simulink model "Project_SADC"  (R2021b)
settings: Solver=ode45  StartTime=0.0  StopTime=T  FixedStep=1e-6  RelTol=1e-12
values from neighbouring files (symbols this model uses):
  A = [A_sc,A_sp]    [Main_SADC_10572571.m]
  Abn0 = Anb0'    [Main_SADC_10572571.m]
  epsilon = deg2rad(23.45)    [Main_SADC_10572571.m]
  m = [0.01 0.05 0.01]'    [Main_SADC_10572571.m]
  N = [n1 n2 n3 n4 n5 n6 n7 n8 n9 n10]    [Main_SADC_10572571.m]
  n_sun = 2*pi / T_sun    (= 1.99238499086e-07)    [Main_SADC_10572571.m]
  P_srp = Fe_tot/c    [Main_SADC_10572571.m]
  R3H0 = data.Re^3*H0    [Main_SADC_10572571.m]
  R_sun = astroConstants(2)    [Main_SADC_10572571.m]
  rho_d = cat(2,ones(1,6)*rho_d_sc,ones(1,4)*rho_d_sp)    [Main_SADC_10572571.m]
  rho_s = cat(2,ones(1,6)*rho_s_sc,ones(1,4)*rho_s_sp)    [Main_SADC_10572571.m]
  ri = [ri_sc,r_sp1,r_sp1,r_sp2,r_sp2]    [Main_SADC_10572571.m]
  w0 = [wx0 wy0 wz0]'    [Main_SADC_10572571.m]
  weights = [0.15;0.5;0.35]    [Main_SADC_10572571.m]
undefined symbols (not defined in the file or in its folder): data, gyro, horizonsensor, magnetometer, rr0, sc, sunsensor, vv0, wheel
libraries: simulink_extras x10
(part 3 of 3)

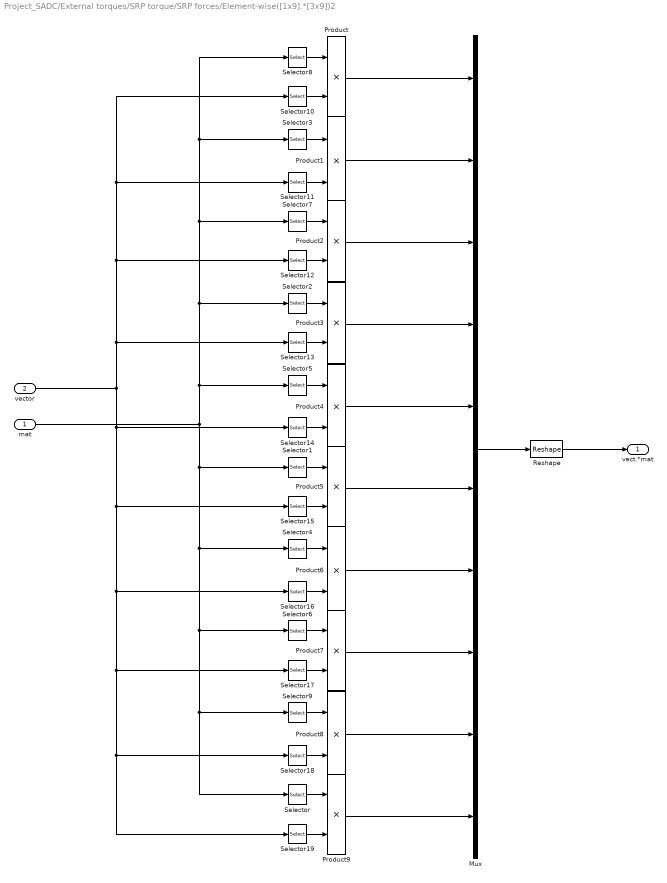
== system Project_SADC/External torques/SRP torque/SRP forces/Element-wise([1x9].*[3x9])2 ==
  mat : Inport
  vector : Inport  Port=2
  Mux : Mux  Inputs=10
  Product{,1..9} (10 alike) : Product
  Reshape : Reshape  OutputDimensionality=Customize  OutputDimensions=[3,10]
  Selector : Selector  NumberOfDimensions=2  InputPortWidth=3  IndexOptions=Index vector (dialog),Index vector (dialog)  Indices=[1 2 3],10  OutputSizes=1,1
  Selector1 : Selector  NumberOfDimensions=2  InputPortWidth=3  IndexOptions=Index vector (dialog),Index vector (dialog)  Indices=[1 2 3],6  OutputSizes=1,1
  Selector10 : Selector  InputPortWidth=10  IndexOptions=Index vector (dialog)  Indices=1  OutputSizes=1
  Selector11 : Selector  InputPortWidth=10  IndexOptions=Index vector (dialog)  Indices=2  OutputSizes=1
  Selector12 : Selector  InputPortWidth=10  IndexOptions=Index vector (dialog)  Indices=3  OutputSizes=1
  Selector13 : Selector  InputPortWidth=10  IndexOptions=Index vector (dialog)  Indices=4  OutputSizes=1
  Selector14 : Selector  InputPortWidth=10  IndexOptions=Index vector (dialog)  Indices=5  OutputSizes=1
  Selector15 : Selector  InputPortWidth=10  IndexOptions=Index vector (dialog)  Indices=6  OutputSizes=1
  Selector16 : Selector  InputPortWidth=10  IndexOptions=Index vector (dialog)  Indices=7  OutputSizes=1
  Selector17 : Selector  InputPortWidth=10  IndexOptions=Index vector (dialog)  Indices=8  OutputSizes=1
  Selector18 : Selector  InputPortWidth=10  IndexOptions=Index vector (dialog)  Indices=9  OutputSizes=1
  Selector19 : Selector  InputPortWidth=10  IndexOptions=Index vector (dialog)  Indices=10  OutputSizes=1
  Selector2 : Selector  NumberOfDimensions=2  InputPortWidth=3  IndexOptions=Index vector (dialog),Index vector (dialog)  Indices=[1 2 3],4  OutputSizes=1,1
  Selector3 : Selector  NumberOfDimensions=2  InputPortWidth=3  IndexOptions=Index vector (dialog),Index vector (dialog)  Indices=[1 2 3],2  OutputSizes=1,1
  Selector4 : Selector  NumberOfDimensions=2  InputPortWidth=3  IndexOptions=Index vector (dialog),Index vector (dialog)  Indices=[1 2 3],7  OutputSizes=1,1
  Selector5 : Selector  NumberOfDimensions=2  InputPortWidth=3  IndexOptions=Index vector (dialog),Index vector (dialog)  Indices=[1 2 3],5  OutputSizes=1,1
  Selector6 : Selector  NumberOfDimensions=2  InputPortWidth=3  IndexOptions=Index vector (dialog),Index vector (dialog)  Indices=[1 2 3],8  OutputSizes=1,1
  Selector7 : Selector  NumberOfDimensions=2  InputPortWidth=3  IndexOptions=Index vector (dialog),Index vector (dialog)  Indices=[1 2 3],3  OutputSizes=1,1
  Selector8 : Selector  NumberOfDimensions=2  InputPortWidth=3  IndexOptions=Index vector (dialog),Index vector (dialog)  Indices=[1 2 3],1  OutputSizes=1,1
  Selector9 : Selector  NumberOfDimensions=2  InputPortWidth=3  IndexOptions=Index vector (dialog),Index vector (dialog)  Indices=[1 2 3],9  OutputSizes=1,1
  vect.*mat : Outport
  wires:
  Product/1 -> Mux/1
  Product1/1 -> Mux/2
  Product2/1 -> Mux/3
  Product3/1 -> Mux/4
  Product4/1 -> Mux/5
  Product6/1 -> Mux/7
  Product5/1 -> Mux/6
  Product7/1 -> Mux/8
  Product8/1 -> Mux/9
  Product9/1 -> Mux/10
  Selector3/1 -> Product1/1
  Selector11/1 -> Product1/2
  Selector7/1 -> Product2/1
  Selector12/1 -> Product2/2
  Selector2/1 -> Product3/1
  Selector13/1 -> Product3/2
  Selector5/1 -> Product4/1
  Selector14/1 -> Product4/2
  Selector1/1 -> Product5/1
  Selector15/1 -> Product5/2
  Selector4/1 -> Product6/1
  Selector16/1 -> Product6/2
  Selector6/1 -> Product7/1
  Selector17/1 -> Product7/2
  Selector18/1 -> Product8/2
  Selector9/1 -> Product8/1
  Selector19/1 -> Product9/2
  Selector/1 -> Product9/1
  Selector10/1 -> Product/2
  Selector8/1 -> Product/1
  vector/1 -> Selector10/1, Selector11/1, Selector12/1, Selector13/1, Selector14/1, Selector15/1, Selector16/1, Selector17/1, Selector18/1, Selector19/1
  mat/1 -> Selector9/1, Selector/1, Selector6/1, Selector4/1, Selector1/1, Selector8/1, Selector3/1, Selector7/1, Selector2/1, Selector5/1
  Reshape/1 -> vect.*mat/1
  Mux/1 -> Reshape/1

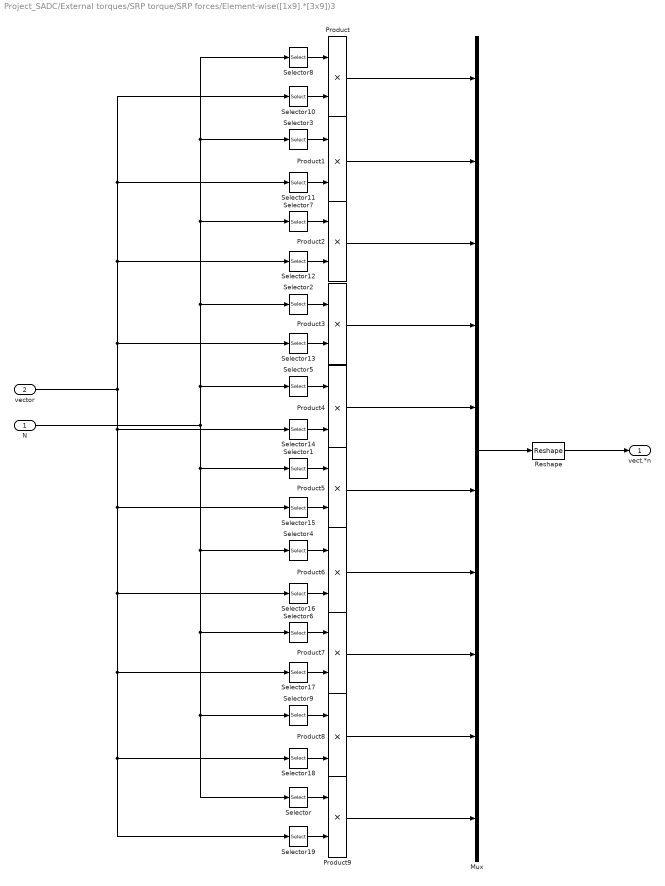
== system Project_SADC/External torques/SRP torque/SRP forces/Element-wise([1x9].*[3x9])3 ==
  N : Inport
  vector : Inport  Port=2
  Mux : Mux  Inputs=10
  Product{,1..9} (10 alike) : Product
  Reshape : Reshape  OutputDimensionality=Customize  OutputDimensions=[3,10]
  Selector : Selector  NumberOfDimensions=2  InputPortWidth=3  IndexOptions=Index vector (dialog),Index vector (dialog)  Indices=[1 2 3],10  OutputSizes=1,1
  Selector1 : Selector  NumberOfDimensions=2  InputPortWidth=3  IndexOptions=Index vector (dialog),Index vector (dialog)  Indices=[1 2 3],6  OutputSizes=1,1
  Selector10 : Selector  InputPortWidth=10  IndexOptions=Index vector (dialog)  Indices=1  OutputSizes=1
  Selector11 : Selector  InputPortWidth=10  IndexOptions=Index vector (dialog)  Indices=2  OutputSizes=1
  Selector12 : Selector  InputPortWidth=10  IndexOptions=Index vector (dialog)  Indices=3  OutputSizes=1
  Selector13 : Selector  InputPortWidth=10  IndexOptions=Index vector (dialog)  Indices=4  OutputSizes=1
  Selector14 : Selector  InputPortWidth=10  IndexOptions=Index vector (dialog)  Indices=5  OutputSizes=1
  Selector15 : Selector  InputPortWidth=10  IndexOptions=Index vector (dialog)  Indices=6  OutputSizes=1
  Selector16 : Selector  InputPortWidth=10  IndexOptions=Index vector (dialog)  Indices=7  OutputSizes=1
  Selector17 : Selector  InputPortWidth=10  IndexOptions=Index vector (dialog)  Indices=8  OutputSizes=1
  Selector18 : Selector  InputPortWidth=10  IndexOptions=Index vector (dialog)  Indices=9  OutputSizes=1
  Selector19 : Selector  InputPortWidth=10  IndexOptions=Index vector (dialog)  Indices=10  OutputSizes=1
  Selector2 : Selector  NumberOfDimensions=2  InputPortWidth=3  IndexOptions=Index vector (dialog),Index vector (dialog)  Indices=[1 2 3],4  OutputSizes=1,1
  Selector3 : Selector  NumberOfDimensions=2  InputPortWidth=3  IndexOptions=Index vector (dialog),Index vector (dialog)  Indices=[1 2 3],2  OutputSizes=1,1
  Selector4 : Selector  NumberOfDimensions=2  InputPortWidth=3  IndexOptions=Index vector (dialog),Index vector (dialog)  Indices=[1 2 3],7  OutputSizes=1,1
  Selector5 : Selector  NumberOfDimensions=2  InputPortWidth=3  IndexOptions=Index vector (dialog),Index vector (dialog)  Indices=[1 2 3],5  OutputSizes=1,1
  Selector6 : Selector  NumberOfDimensions=2  InputPortWidth=3  IndexOptions=Index vector (dialog),Index vector (dialog)  Indices=[1 2 3],8  OutputSizes=1,1
  Selector7 : Selector  NumberOfDimensions=2  InputPortWidth=3  IndexOptions=Index vector (dialog),Index vector (dialog)  Indices=[1 2 3],3  OutputSizes=1,1
  Selector8 : Selector  NumberOfDimensions=2  InputPortWidth=3  IndexOptions=Index vector (dialog),Index vector (dialog)  Indices=[1 2 3],1  OutputSizes=1,1
  Selector9 : Selector  NumberOfDimensions=2  InputPortWidth=3  IndexOptions=Index vector (dialog),Index vector (dialog)  Indices=[1 2 3],9  OutputSizes=1,1
  vect.*n : Outport
  wires:
  Product/1 -> Mux/1
  Product1/1 -> Mux/2
  Product2/1 -> Mux/3
  Product3/1 -> Mux/4
  Product4/1 -> Mux/5
  Product6/1 -> Mux/7
  Product5/1 -> Mux/6
  Product7/1 -> Mux/8
  Product8/1 -> Mux/9
  Product9/1 -> Mux/10
  Selector3/1 -> Product1/1
  Selector11/1 -> Product1/2
  Selector7/1 -> Product2/1
  Selector12/1 -> Product2/2
  Selector2/1 -> Product3/1
  Selector13/1 -> Product3/2
  Selector5/1 -> Product4/1
  Selector14/1 -> Product4/2
  Selector1/1 -> Product5/1
  Selector15/1 -> Product5/2
  Selector4/1 -> Product6/1
  Selector16/1 -> Product6/2
  Selector6/1 -> Product7/1
  Selector17/1 -> Product7/2
  Selector18/1 -> Product8/2
  Selector9/1 -> Product8/1
  Selector19/1 -> Product9/2
  Selector/1 -> Product9/1
  Selector10/1 -> Product/2
  Selector8/1 -> Product/1
  vector/1 -> Selector10/1, Selector11/1, Selector12/1, Selector13/1, Selector14/1, Selector15/1, Selector16/1, Selector17/1, Selector18/1, Selector19/1
  N/1 -> Selector9/1, Selector/1, Selector6/1, Selector4/1, Selector1/1, Selector8/1, Selector3/1, Selector7/1, Selector2/1, Selector5/1
  Reshape/1 -> vect.*n/1
  Mux/1 -> Reshape/1

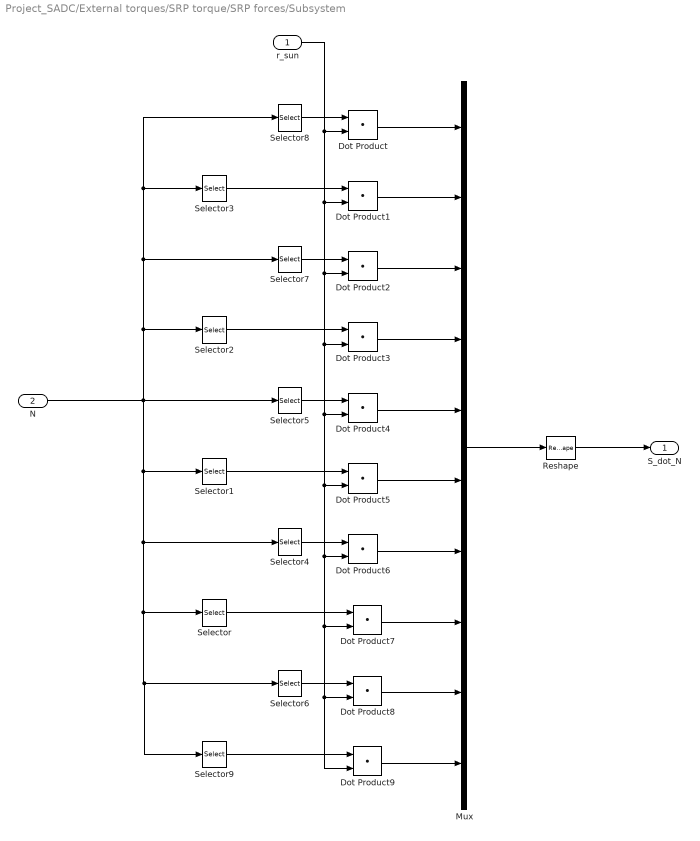
== system Project_SADC/External torques/SRP torque/SRP forces/Subsystem ==
  r_sun : Inport
  N : Inport  Port=2
  Dot Product{,1..9} (10 alike) : DotProduct  InputSameDT=on  OutDataTypeStr=Inherit: Inherit via internal rule
  Mux : Mux  Inputs=10
  Reshape : Reshape  OutputDimensionality=Row vector (2-D)
  Selector : Selector  NumberOfDimensions=2  InputPortWidth=3  IndexOptions=Index vector (dialog),Index vector (dialog)  Indices=[1 2 3],8  OutputSizes=1,1
  Selector1 : Selector  NumberOfDimensions=2  InputPortWidth=3  IndexOptions=Index vector (dialog),Index vector (dialog)  Indices=[1 2 3],6  OutputSizes=1,1
  Selector2 : Selector  NumberOfDimensions=2  InputPortWidth=3  IndexOptions=Index vector (dialog),Index vector (dialog)  Indices=[1 2 3],4  OutputSizes=1,1
  Selector3 : Selector  NumberOfDimensions=2  InputPortWidth=3  IndexOptions=Index vector (dialog),Index vector (dialog)  Indices=[1 2 3],2  OutputSizes=1,1
  Selector4 : Selector  NumberOfDimensions=2  InputPortWidth=3  IndexOptions=Index vector (dialog),Index vector (dialog)  Indices=[1 2 3],7  OutputSizes=1,1
  Selector5 : Selector  NumberOfDimensions=2  InputPortWidth=3  IndexOptions=Index vector (dialog),Index vector (dialog)  Indices=[1 2 3],5  OutputSizes=1,1
  Selector6 : Selector  NumberOfDimensions=2  InputPortWidth=3  IndexOptions=Index vector (dialog),Index vector (dialog)  Indices=[1 2 3],9  OutputSizes=1,1
  Selector7 : Selector  NumberOfDimensions=2  InputPortWidth=3  IndexOptions=Index vector (dialog),Index vector (dialog)  Indices=[1 2 3],3  OutputSizes=1,1
  Selector8 : Selector  NumberOfDimensions=2  InputPortWidth=3  IndexOptions=Index vector (dialog),Index vector (dialog)  Indices=[1 2 3],1  OutputSizes=1,1
  Selector9 : Selector  NumberOfDimensions=2  InputPortWidth=3  IndexOptions=Index vector (dialog),Index vector (dialog)  Indices=[1 2 3],10  OutputSizes=1,1
  S_dot_N : Outport
  wires:
  N/1 -> Selector9/1, Selector6/1, Selector/1, Selector4/1, Selector1/1, Selector7/1, Selector8/1, Selector3/1, Selector2/1, Selector5/1
  Selector8/1 -> Dot Product/1
  Selector3/1 -> Dot Product1/1
  Selector7/1 -> Dot Product2/1
  Selector2/1 -> Dot Product3/1
  Selector5/1 -> Dot Product4/1
  Selector1/1 -> Dot Product5/1
  Selector4/1 -> Dot Product6/1
  Selector/1 -> Dot Product7/1
  Selector6/1 -> Dot Product8/1
  Selector9/1 -> Dot Product9/1
  r_sun/1 -> Dot Product9/2, Dot Product8/2, Dot Product7/2, Dot Product6/2, Dot Product5/2, Dot Product4/2, Dot Product3/2, Dot Product2/2, Dot Product1/2, Dot Product/2
  Dot Product/1 -> Mux/1
  Dot Product9/1 -> Mux/10
  Dot Product8/1 -> Mux/9
  Dot Product7/1 -> Mux/8
  Dot Product6/1 -> Mux/7
  Dot Product5/1 -> Mux/6
  Dot Product4/1 -> Mux/5
  Dot Product3/1 -> Mux/4
  Dot Product1/1 -> Mux/2
  Dot Product2/1 -> Mux/3
  Mux/1 -> Reshape/1
  Reshape/1 -> S_dot_N/1

== system Project_SADC/External torques/SRP torque/SRP forces/Vector norm1 ==
  u : Inport
  Divide : Product  Inputs=*/
  norm_vector : Subsystem
  u_versor : Outport
  ||u|| : Outport  Port=2
  wires:
  u/1 -> Divide/1, norm_vector/1(u)
  norm_vector/1(|u|) -> ||u||/1, Divide/2
  Divide/1 -> u_versor/1

== system Project_SADC/External torques/SRP torque/Sun wrt s//c/R_Sun in inertial ==
  t : Inport
  Constant1 : Constant  Value=n_sun
  Constant2 : Constant  Value=epsilon
  Constant3 : Constant  Value=epsilon
  Cos : Trigonometry  Operator=cos
  Cos1 : Trigonometry  Operator=cos
  Gain : Gain  Gain=R_sun
  Mux : Mux  Inputs=3
  Product : Product
  Product1 : Product
  Product2 : Product
  Reshape : Reshape  OutputDimensionality=Column vector (2-D)
  Sin : Trigonometry
  Sin1 : Trigonometry
  Sin2 : Trigonometry
  R_sun_N : Outport
  wires:
  t/1 -> Product/2
  Constant1/1 -> Product/1
  Product/1 -> Sin1/1, Sin2/1, Cos/1
  Constant2/1 -> Cos1/1
  Constant3/1 -> Sin/1
  Cos1/1 -> Product1/1
  Sin2/1 -> Product1/2
  Sin/1 -> Product2/1
  Sin1/1 -> Product2/2
  Product1/1 -> Mux/2
  Product2/1 -> Mux/3
  Cos/1 -> Mux/1
  Mux/1 -> Reshape/1
  Gain/1 -> R_sun_N/1
  Reshape/1 -> Gain/1

== system Project_SADC/External torques/SRP torque/Torques on faces of s//c/product vector ==
  A : Inport
  B : Inport  Port=2
  Mux : Mux  Inputs=3
  i-component : Subsystem
  j-component : Subsystem
  k-component1 : Subsystem
  C : Outport
  wires:
  Mux/1 -> C/1
  A/1 -> k-component1/1(A), j-component/1(A), i-component/1(A)
  B/1 -> k-component1/2(B), j-component/2(B), i-component/2(B)
  i-component/1(Out2) -> Mux/1
  j-component/1(Out1) -> Mux/2
  k-component1/1(Out1) -> Mux/3

== system Project_SADC/External torques/SRP torque/Torques on faces of s//c/product vector1 ==
  A : Inport
  B : Inport  Port=2
  Mux : Mux  Inputs=3
  i-component : Subsystem
  j-component : Subsystem
  k-component1 : Subsystem
  C : Outport
  wires:
  k-component1/1(Out1) -> Mux/3
  j-component/1(Out1) -> Mux/2
  i-component/1(Out2) -> Mux/1
  B/1 -> i-component/2(B), j-component/2(B), k-component1/2(B)
  A/1 -> i-component/1(A), j-component/1(A), k-component1/1(A)
  Mux/1 -> C/1

== system Project_SADC/External torques/SRP torque/Torques on faces of s//c/product vector2 ==
  A : Inport
  B : Inport  Port=2
  Mux : Mux  Inputs=3
  i-component : Subsystem
  j-component : Subsystem
  k-component1 : Subsystem
  C : Outport
  wires:
  k-component1/1(Out1) -> Mux/3
  j-component/1(Out1) -> Mux/2
  i-component/1(Out2) -> Mux/1
  B/1 -> i-component/2(B), j-component/2(B), k-component1/2(B)
  A/1 -> i-component/1(A), j-component/1(A), k-component1/1(A)
  Mux/1 -> C/1

== system Project_SADC/External torques/SRP torque/Torques on faces of s//c/product vector3 ==
  A : Inport
  B : Inport  Port=2
  Mux : Mux  Inputs=3
  i-component : Subsystem
  j-component : Subsystem
  k-component1 : Subsystem
  C : Outport
  wires:
  Mux/1 -> C/1
  A/1 -> k-component1/1(A), j-component/1(A), i-component/1(A)
  B/1 -> k-component1/2(B), j-component/2(B), i-component/2(B)
  i-component/1(Out2) -> Mux/1
  j-component/1(Out1) -> Mux/2
  k-component1/1(Out1) -> Mux/3

== system Project_SADC/External torques/SRP torque/Torques on faces of s//c/product vector4 ==
  A : Inport
  B : Inport  Port=2
  Mux : Mux  Inputs=3
  i-component : Subsystem
  j-component : Subsystem
  k-component1 : Subsystem
  C : Outport
  wires:
  k-component1/1(Out1) -> Mux/3
  j-component/1(Out1) -> Mux/2
  i-component/1(Out2) -> Mux/1
  B/1 -> i-component/2(B), j-component/2(B), k-component1/2(B)
  A/1 -> i-component/1(A), j-component/1(A), k-component1/1(A)
  Mux/1 -> C/1

== system Project_SADC/External torques/SRP torque/Torques on faces of s//c/product vector5 ==
  A : Inport
  B : Inport  Port=2
  Mux : Mux  Inputs=3
  i-component : Subsystem
  j-component : Subsystem
  k-component1 : Subsystem
  C : Outport
  wires:
  Mux/1 -> C/1
  A/1 -> k-component1/1(A), j-component/1(A), i-component/1(A)
  B/1 -> k-component1/2(B), j-component/2(B), i-component/2(B)
  i-component/1(Out2) -> Mux/1
  j-component/1(Out1) -> Mux/2
  k-component1/1(Out1) -> Mux/3

== system Project_SADC/External torques/SRP torque/Torques on faces of s//c/product vector6 ==
  A : Inport
  B : Inport  Port=2
  Mux : Mux  Inputs=3
  i-component : Subsystem
  j-component : Subsystem
  k-component1 : Subsystem
  C : Outport
  wires:
  k-component1/1(Out1) -> Mux/3
  j-component/1(Out1) -> Mux/2
  i-component/1(Out2) -> Mux/1
  B/1 -> i-component/2(B), j-component/2(B), k-component1/2(B)
  A/1 -> i-component/1(A), j-component/1(A), k-component1/1(A)
  Mux/1 -> C/1

== system Project_SADC/External torques/SRP torque/Torques on faces of s//c/product vector7 ==
  A : Inport
  B : Inport  Port=2
  Mux : Mux  Inputs=3
  i-component : Subsystem
  j-component : Subsystem
  k-component1 : Subsystem
  C : Outport
  wires:
  Mux/1 -> C/1
  A/1 -> k-component1/1(A), j-component/1(A), i-component/1(A)
  B/1 -> k-component1/2(B), j-component/2(B), i-component/2(B)
  i-component/1(Out2) -> Mux/1
  j-component/1(Out1) -> Mux/2
  k-component1/1(Out1) -> Mux/3

== system Project_SADC/External torques/SRP torque/Torques on faces of s//c/product vector8 ==
  A : Inport
  B : Inport  Port=2
  Mux : Mux  Inputs=3
  i-component : Subsystem
  j-component : Subsystem
  k-component1 : Subsystem
  C : Outport
  wires:
  k-component1/1(Out1) -> Mux/3
  j-component/1(Out1) -> Mux/2
  i-component/1(Out2) -> Mux/1
  B/1 -> i-component/2(B), j-component/2(B), k-component1/2(B)
  A/1 -> i-component/1(A), j-component/1(A), k-component1/1(A)
  Mux/1 -> C/1

== system Project_SADC/External torques/SRP torque/Torques on faces of s//c/product vector9 ==
  A : Inport
  B : Inport  Port=2
  Mux : Mux  Inputs=3
  i-component : Subsystem
  j-component : Subsystem
  k-component1 : Subsystem
  C : Outport
  wires:
  Mux/1 -> C/1
  A/1 -> k-component1/1(A), j-component/1(A), i-component/1(A)
  B/1 -> k-component1/2(B), j-component/2(B), i-component/2(B)
  i-component/1(Out2) -> Mux/1
  j-component/1(Out1) -> Mux/2
  k-component1/1(Out1) -> Mux/3

== system Project_SADC/Orbit/Orbit integration /Subsystem1/norm_vector ==
  u : Inport
  Demux : Demux  Outputs=3
  Square : Math  Operator=square  SaturateOnIntegerOverflow=on
  Square Root : Sqrt  SaturateOnIntegerOverflow=on
  Square1 : Math  Operator=square  SaturateOnIntegerOverflow=on
  Square3 : Math  Operator=square  SaturateOnIntegerOverflow=on
  Sum : Sum  Inputs=+++
  |u| : Outport
  wires:
  u/1 -> Demux/1
  Demux/1 -> Square/1
  Demux/2 -> Square1/1
  Demux/3 -> Square3/1
  Square/1 -> Sum/1
  Square3/1 -> Sum/3
  Square1/1 -> Sum/2
  Sum/1 -> Square Root/1
  Square Root/1 -> |u|/1

== system Project_SADC/Relative Attitude/DCM from L to B and from L to N/DCM from L to N/Vector norm ==
  u : Inport
  Divide : Product  Inputs=*/
  norm_vector : Subsystem
  u_versor : Outport
  ||u|| : Outport  Port=2
  wires:
  u/1 -> Divide/1, norm_vector/1(u)
  norm_vector/1(|u|) -> ||u||/1, Divide/2
  Divide/1 -> u_versor/1

== system Project_SADC/Relative Attitude/DCM from L to B and from L to N/DCM from L to N/Vector norm1 ==
  u : Inport
  Divide : Product  Inputs=*/
  norm_vector : Subsystem
  u_versor : Outport
  ||u|| : Outport  Port=2
  wires:
  u/1 -> Divide/1, norm_vector/1(u)
  norm_vector/1(|u|) -> ||u||/1, Divide/2
  Divide/1 -> u_versor/1

== system Project_SADC/Relative Attitude/DCM from L to B and from L to N/DCM from L to N/product vector ==
  A : Inport
  B : Inport  Port=2
  Mux : Mux  Inputs=3
  i-component : Subsystem
  j-component : Subsystem
  k-component1 : Subsystem
  C : Outport
  wires:
  Mux/1 -> C/1
  A/1 -> k-component1/1(A), j-component/1(A), i-component/1(A)
  B/1 -> k-component1/2(B), j-component/2(B), i-component/2(B)
  i-component/1(Out2) -> Mux/1
  j-component/1(Out1) -> Mux/2
  k-component1/1(Out1) -> Mux/3

== system Project_SADC/Relative Attitude/DCM from L to B and from L to N/Vector norm/norm_vector ==
  u : Inport
  Demux : Demux  Outputs=3
  Square : Math  Operator=square  SaturateOnIntegerOverflow=on
  Square Root : Sqrt  SaturateOnIntegerOverflow=on
  Square1 : Math  Operator=square  SaturateOnIntegerOverflow=on
  Square3 : Math  Operator=square  SaturateOnIntegerOverflow=on
  Sum : Sum  Inputs=+++
  |u| : Outport
  wires:
  u/1 -> Demux/1
  Demux/1 -> Square/1
  Demux/2 -> Square1/1
  Demux/3 -> Square3/1
  Square/1 -> Sum/1
  Square3/1 -> Sum/3
  Square1/1 -> Sum/2
  Sum/1 -> Square Root/1
  Square Root/1 -> |u|/1

== system Project_SADC/Relative Attitude/DCM from L to B and from L to N/Vector norm1/norm_vector ==
  u : Inport
  Demux : Demux  Outputs=3
  Square : Math  Operator=square  SaturateOnIntegerOverflow=on
  Square Root : Sqrt  SaturateOnIntegerOverflow=on
  Square1 : Math  Operator=square  SaturateOnIntegerOverflow=on
  Square3 : Math  Operator=square  SaturateOnIntegerOverflow=on
  Sum : Sum  Inputs=+++
  |u| : Outport
  wires:
  Square Root/1 -> |u|/1
  Sum/1 -> Square Root/1
  Square1/1 -> Sum/2
  Square3/1 -> Sum/3
  Square/1 -> Sum/1
  Demux/3 -> Square3/1
  Demux/2 -> Square1/1
  Demux/1 -> Square/1
  u/1 -> Demux/1

== system Project_SADC/Sensors/Check if in EH FOV/Vector norm1/norm_vector ==
  u : Inport
  Demux : Demux  Outputs=3
  Square : Math  Operator=square  SaturateOnIntegerOverflow=on
  Square Root : Sqrt  SaturateOnIntegerOverflow=on
  Square1 : Math  Operator=square  SaturateOnIntegerOverflow=on
  Square3 : Math  Operator=square  SaturateOnIntegerOverflow=on
  Sum : Sum  Inputs=+++
  |u| : Outport
  wires:
  u/1 -> Demux/1
  Demux/1 -> Square/1
  Demux/2 -> Square1/1
  Demux/3 -> Square3/1
  Square/1 -> Sum/1
  Square3/1 -> Sum/3
  Square1/1 -> Sum/2
  Sum/1 -> Square Root/1
  Square Root/1 -> |u|/1

== system Project_SADC/Sensors/Check if in sunsensor FOV/Vector norm1/norm_vector ==
  u : Inport
  Demux : Demux  Outputs=3
  Square : Math  Operator=square  SaturateOnIntegerOverflow=on
  Square Root : Sqrt  SaturateOnIntegerOverflow=on
  Square1 : Math  Operator=square  SaturateOnIntegerOverflow=on
  Square3 : Math  Operator=square  SaturateOnIntegerOverflow=on
  Sum : Sum  Inputs=+++
  |u| : Outport
  wires:
  Square Root/1 -> |u|/1
  Sum/1 -> Square Root/1
  Square1/1 -> Sum/2
  Square3/1 -> Sum/3
  Square/1 -> Sum/1
  Demux/3 -> Square3/1
  Demux/2 -> Square1/1
  Demux/1 -> Square/1
  u/1 -> Demux/1

== system Project_SADC/Sensors/Cylindrical eclipse model/Vec tor norm2/norm_vector ==
  u : Inport
  Demux : Demux  Outputs=3
  Square : Math  Operator=square  SaturateOnIntegerOverflow=on
  Square Root : Sqrt  SaturateOnIntegerOverflow=on
  Square1 : Math  Operator=square  SaturateOnIntegerOverflow=on
  Square3 : Math  Operator=square  SaturateOnIntegerOverflow=on
  Sum : Sum  Inputs=+++
  |u| : Outport
  wires:
  u/1 -> Demux/1
  Demux/1 -> Square/1
  Demux/2 -> Square1/1
  Demux/3 -> Square3/1
  Square/1 -> Sum/1
  Square3/1 -> Sum/3
  Square1/1 -> Sum/2
  Sum/1 -> Square Root/1
  Square Root/1 -> |u|/1

== system Project_SADC/Sensors/Cylindrical eclipse model/Vector norm1/norm_vector ==
  u : Inport
  Demux : Demux  Outputs=3
  Square : Math  Operator=square  SaturateOnIntegerOverflow=on
  Square Root : Sqrt  SaturateOnIntegerOverflow=on
  Square1 : Math  Operator=square  SaturateOnIntegerOverflow=on
  Square3 : Math  Operator=square  SaturateOnIntegerOverflow=on
  Sum : Sum  Inputs=+++
  |u| : Outport
  wires:
  Square Root/1 -> |u|/1
  Sum/1 -> Square Root/1
  Square1/1 -> Sum/2
  Square3/1 -> Sum/3
  Square/1 -> Sum/1
  Demux/3 -> Square3/1
  Demux/2 -> Square1/1
  Demux/1 -> Square/1
  u/1 -> Demux/1

== system Project_SADC/Sensors/Cylindrical eclipse model/Vector norm2/norm_vector ==
  u : Inport
  Demux : Demux  Outputs=3
  Square : Math  Operator=square  SaturateOnIntegerOverflow=on
  Square Root : Sqrt  SaturateOnIntegerOverflow=on
  Square1 : Math  Operator=square  SaturateOnIntegerOverflow=on
  Square3 : Math  Operator=square  SaturateOnIntegerOverflow=on
  Sum : Sum  Inputs=+++
  |u| : Outport
  wires:
  u/1 -> Demux/1
  Demux/1 -> Square/1
  Demux/2 -> Square1/1
  Demux/3 -> Square3/1
  Square/1 -> Sum/1
  Square3/1 -> Sum/3
  Square1/1 -> Sum/2
  Sum/1 -> Square Root/1
  Square Root/1 -> |u|/1

== system Project_SADC/Sensors/Cylindrical eclipse model/Vector norm3/norm_vector ==
  u : Inport
  Demux : Demux  Outputs=3
  Square : Math  Operator=square  SaturateOnIntegerOverflow=on
  Square Root : Sqrt  SaturateOnIntegerOverflow=on
  Square1 : Math  Operator=square  SaturateOnIntegerOverflow=on
  Square3 : Math  Operator=square  SaturateOnIntegerOverflow=on
  Sum : Sum  Inputs=+++
  |u| : Outport
  wires:
  Square Root/1 -> |u|/1
  Sum/1 -> Square Root/1
  Square1/1 -> Sum/2
  Square3/1 -> Sum/3
  Square/1 -> Sum/1
  Demux/3 -> Square3/1
  Demux/2 -> Square1/1
  Demux/1 -> Square/1
  u/1 -> Demux/1

== system Project_SADC/External torques/Magnetic torque/mag_field in inertial/Vector norm1/norm_vector ==
  u : Inport
  Demux : Demux  Outputs=3
  Square : Math  Operator=square  SaturateOnIntegerOverflow=on
  Square Root : Sqrt  SaturateOnIntegerOverflow=on
  Square1 : Math  Operator=square  SaturateOnIntegerOverflow=on
  Square3 : Math  Operator=square  SaturateOnIntegerOverflow=on
  Sum : Sum  Inputs=+++
  |u| : Outport
  wires:
  u/1 -> Demux/1
  Demux/1 -> Square/1
  Demux/2 -> Square1/1
  Demux/3 -> Square3/1
  Square/1 -> Sum/1
  Square3/1 -> Sum/3
  Square1/1 -> Sum/2
  Sum/1 -> Square Root/1
  Square Root/1 -> |u|/1

== system Project_SADC/External torques/SRP torque/SRP forces/Vector norm1/norm_vector ==
  u : Inport
  Demux : Demux  Outputs=3
  Square : Math  Operator=square  SaturateOnIntegerOverflow=on
  Square Root : Sqrt  SaturateOnIntegerOverflow=on
  Square1 : Math  Operator=square  SaturateOnIntegerOverflow=on
  Square3 : Math  Operator=square  SaturateOnIntegerOverflow=on
  Sum : Sum  Inputs=+++
  |u| : Outport
  wires:
  u/1 -> Demux/1
  Demux/1 -> Square/1
  Demux/2 -> Square1/1
  Demux/3 -> Square3/1
  Square/1 -> Sum/1
  Square3/1 -> Sum/3
  Square1/1 -> Sum/2
  Sum/1 -> Square Root/1
  Square Root/1 -> |u|/1

== system Project_SADC/External torques/SRP torque/Torques on faces of s//c/product vector/i-component ==
  A : Inport
  B : Inport  Port=2
  Demux : Demux  Outputs=3
  Demux1 : Demux  Outputs=3
  Product : Product
  Product1 : Product
  Sum : Sum  Inputs=+-
  Terminator : Terminator
  Terminator1 : Terminator
  Out2 : Outport
  wires:
  Sum/1 -> Out2/1
  Product1/1 -> Sum/2  "a3b2"
  Demux1/2 -> Product1/2  "b2"
  Product/1 -> Sum/1  "a2b3"
  Demux/2 -> Product/1  "a2"
  Demux/3 -> Product1/1  "a3"
  Demux1/3 -> Product/2  "b3"
  Demux/1 -> Terminator/1  "a1"
  Demux1/1 -> Terminator1/1
  B/1 -> Demux1/1
  A/1 -> Demux/1

== system Project_SADC/External torques/SRP torque/Torques on faces of s//c/product vector/j-component ==
  A : Inport
  B : Inport  Port=2
  Demux : Demux  Outputs=3
  Demux1 : Demux  Outputs=3
  Product : Product
  Product1 : Product
  Sum : Sum  Inputs=+-
  Terminator : Terminator
  Terminator1 : Terminator
  Out1 : Outport
  wires:
  B/1 -> Demux1/1
  A/1 -> Demux/1
  Demux/3 -> Product/1  "a3"
  Demux1/1 -> Product/2  "b1"
  Demux/1 -> Product1/1  "a1"
  Demux1/3 -> Product1/2  "b3"
  Demux1/2 -> Terminator/1
  Demux/2 -> Terminator1/1
  Product/1 -> Sum/1
  Product1/1 -> Sum/2
  Sum/1 -> Out1/1

== system Project_SADC/External torques/SRP torque/Torques on faces of s//c/product vector/k-component1 ==
  A : Inport
  B : Inport  Port=2
  Demux : Demux  Outputs=3
  Demux1 : Demux  Outputs=3
  Product : Product
  Product1 : Product
  Sum : Sum  Inputs=+-
  Terminator : Terminator
  Terminator1 : Terminator
  Out1 : Outport
  wires:
  Sum/1 -> Out1/1
  Product1/1 -> Sum/2
  Product/1 -> Sum/1
  Demux1/2 -> Product/2  "b2"
  A/1 -> Demux/1
  B/1 -> Demux1/1
  Demux/1 -> Product/1  "a1"
  Demux/2 -> Product1/1  "a2"
  Demux1/1 -> Product1/2  "b1"
  Demux1/3 -> Terminator/1  "b3"
  Demux/3 -> Terminator1/1  "a3"

== system Project_SADC/External torques/SRP torque/Torques on faces of s//c/product vector1/i-component ==
  A : Inport
  B : Inport  Port=2
  Demux : Demux  Outputs=3
  Demux1 : Demux  Outputs=3
  Product : Product
  Product1 : Product
  Sum : Sum  Inputs=+-
  Terminator : Terminator
  Terminator1 : Terminator
  Out2 : Outport
  wires:
  A/1 -> Demux/1
  B/1 -> Demux1/1
  Demux1/1 -> Terminator1/1
  Demux/1 -> Terminator/1  "a1"
  Demux1/3 -> Product/2  "b3"
  Demux/3 -> Product1/1  "a3"
  Demux/2 -> Product/1  "a2"
  Product/1 -> Sum/1  "a2b3"
  Demux1/2 -> Product1/2  "b2"
  Product1/1 -> Sum/2  "a3b2"
  Sum/1 -> Out2/1

== system Project_SADC/External torques/SRP torque/Torques on faces of s//c/product vector1/j-component ==
  A : Inport
  B : Inport  Port=2
  Demux : Demux  Outputs=3
  Demux1 : Demux  Outputs=3
  Product : Product
  Product1 : Product
  Sum : Sum  Inputs=+-
  Terminator : Terminator
  Terminator1 : Terminator
  Out1 : Outport
  wires:
  Sum/1 -> Out1/1
  Product1/1 -> Sum/2
  Product/1 -> Sum/1
  Demux/2 -> Terminator1/1
  Demux1/2 -> Terminator/1
  Demux1/3 -> Product1/2  "b3"
  Demux/1 -> Product1/1  "a1"
  Demux1/1 -> Product/2  "b1"
  Demux/3 -> Product/1  "a3"
  A/1 -> Demux/1
  B/1 -> Demux1/1

== system Project_SADC/External torques/SRP torque/Torques on faces of s//c/product vector1/k-component1 ==
  A : Inport
  B : Inport  Port=2
  Demux : Demux  Outputs=3
  Demux1 : Demux  Outputs=3
  Product : Product
  Product1 : Product
  Sum : Sum  Inputs=+-
  Terminator : Terminator
  Terminator1 : Terminator
  Out1 : Outport
  wires:
  Demux/3 -> Terminator1/1  "a3"
  Demux1/3 -> Terminator/1  "b3"
  Demux1/1 -> Product1/2  "b1"
  Demux/2 -> Product1/1  "a2"
  Demux/1 -> Product/1  "a1"
  B/1 -> Demux1/1
  A/1 -> Demux/1
  Demux1/2 -> Product/2  "b2"
  Product/1 -> Sum/1
  Product1/1 -> Sum/2
  Sum/1 -> Out1/1

== system Project_SADC/External torques/SRP torque/Torques on faces of s//c/product vector2/i-component ==
  A : Inport
  B : Inport  Port=2
  Demux : Demux  Outputs=3
  Demux1 : Demux  Outputs=3
  Product : Product
  Product1 : Product
  Sum : Sum  Inputs=+-
  Terminator : Terminator
  Terminator1 : Terminator
  Out2 : Outport
  wires:
  A/1 -> Demux/1
  B/1 -> Demux1/1
  Demux1/1 -> Terminator1/1
  Demux/1 -> Terminator/1  "a1"
  Demux1/3 -> Product/2  "b3"
  Demux/3 -> Product1/1  "a3"
  Demux/2 -> Product/1  "a2"
  Product/1 -> Sum/1  "a2b3"
  Demux1/2 -> Product1/2  "b2"
  Product1/1 -> Sum/2  "a3b2"
  Sum/1 -> Out2/1

== system Project_SADC/External torques/SRP torque/Torques on faces of s//c/product vector2/j-component ==
  A : Inport
  B : Inport  Port=2
  Demux : Demux  Outputs=3
  Demux1 : Demux  Outputs=3
  Product : Product
  Product1 : Product
  Sum : Sum  Inputs=+-
  Terminator : Terminator
  Terminator1 : Terminator
  Out1 : Outport
  wires:
  Sum/1 -> Out1/1
  Product1/1 -> Sum/2
  Product/1 -> Sum/1
  Demux/2 -> Terminator1/1
  Demux1/2 -> Terminator/1
  Demux1/3 -> Product1/2  "b3"
  Demux/1 -> Product1/1  "a1"
  Demux1/1 -> Product/2  "b1"
  Demux/3 -> Product/1  "a3"
  A/1 -> Demux/1
  B/1 -> Demux1/1

== system Project_SADC/External torques/SRP torque/Torques on faces of s//c/product vector2/k-component1 ==
  A : Inport
  B : Inport  Port=2
  Demux : Demux  Outputs=3
  Demux1 : Demux  Outputs=3
  Product : Product
  Product1 : Product
  Sum : Sum  Inputs=+-
  Terminator : Terminator
  Terminator1 : Terminator
  Out1 : Outport
  wires:
  Demux/3 -> Terminator1/1  "a3"
  Demux1/3 -> Terminator/1  "b3"
  Demux1/1 -> Product1/2  "b1"
  Demux/2 -> Product1/1  "a2"
  Demux/1 -> Product/1  "a1"
  B/1 -> Demux1/1
  A/1 -> Demux/1
  Demux1/2 -> Product/2  "b2"
  Product/1 -> Sum/1
  Product1/1 -> Sum/2
  Sum/1 -> Out1/1

== system Project_SADC/External torques/SRP torque/Torques on faces of s//c/product vector3/i-component ==
  A : Inport
  B : Inport  Port=2
  Demux : Demux  Outputs=3
  Demux1 : Demux  Outputs=3
  Product : Product
  Product1 : Product
  Sum : Sum  Inputs=+-
  Terminator : Terminator
  Terminator1 : Terminator
  Out2 : Outport
  wires:
  Sum/1 -> Out2/1
  Product1/1 -> Sum/2  "a3b2"
  Demux1/2 -> Product1/2  "b2"
  Product/1 -> Sum/1  "a2b3"
  Demux/2 -> Product/1  "a2"
  Demux/3 -> Product1/1  "a3"
  Demux1/3 -> Product/2  "b3"
  Demux/1 -> Terminator/1  "a1"
  Demux1/1 -> Terminator1/1
  B/1 -> Demux1/1
  A/1 -> Demux/1

== system Project_SADC/External torques/SRP torque/Torques on faces of s//c/product vector3/j-component ==
  A : Inport
  B : Inport  Port=2
  Demux : Demux  Outputs=3
  Demux1 : Demux  Outputs=3
  Product : Product
  Product1 : Product
  Sum : Sum  Inputs=+-
  Terminator : Terminator
  Terminator1 : Terminator
  Out1 : Outport
  wires:
  B/1 -> Demux1/1
  A/1 -> Demux/1
  Demux/3 -> Product/1  "a3"
  Demux1/1 -> Product/2  "b1"
  Demux/1 -> Product1/1  "a1"
  Demux1/3 -> Product1/2  "b3"
  Demux1/2 -> Terminator/1
  Demux/2 -> Terminator1/1
  Product/1 -> Sum/1
  Product1/1 -> Sum/2
  Sum/1 -> Out1/1

== system Project_SADC/External torques/SRP torque/Torques on faces of s//c/product vector3/k-component1 ==
  A : Inport
  B : Inport  Port=2
  Demux : Demux  Outputs=3
  Demux1 : Demux  Outputs=3
  Product : Product
  Product1 : Product
  Sum : Sum  Inputs=+-
  Terminator : Terminator
  Terminator1 : Terminator
  Out1 : Outport
  wires:
  Sum/1 -> Out1/1
  Product1/1 -> Sum/2
  Product/1 -> Sum/1
  Demux1/2 -> Product/2  "b2"
  A/1 -> Demux/1
  B/1 -> Demux1/1
  Demux/1 -> Product/1  "a1"
  Demux/2 -> Product1/1  "a2"
  Demux1/1 -> Product1/2  "b1"
  Demux1/3 -> Terminator/1  "b3"
  Demux/3 -> Terminator1/1  "a3"

== system Project_SADC/External torques/SRP torque/Torques on faces of s//c/product vector4/i-component ==
  A : Inport
  B : Inport  Port=2
  Demux : Demux  Outputs=3
  Demux1 : Demux  Outputs=3
  Product : Product
  Product1 : Product
  Sum : Sum  Inputs=+-
  Terminator : Terminator
  Terminator1 : Terminator
  Out2 : Outport
  wires:
  A/1 -> Demux/1
  B/1 -> Demux1/1
  Demux1/1 -> Terminator1/1
  Demux/1 -> Terminator/1  "a1"
  Demux1/3 -> Product/2  "b3"
  Demux/3 -> Product1/1  "a3"
  Demux/2 -> Product/1  "a2"
  Product/1 -> Sum/1  "a2b3"
  Demux1/2 -> Product1/2  "b2"
  Product1/1 -> Sum/2  "a3b2"
  Sum/1 -> Out2/1

== system Project_SADC/External torques/SRP torque/Torques on faces of s//c/product vector4/j-component ==
  A : Inport
  B : Inport  Port=2
  Demux : Demux  Outputs=3
  Demux1 : Demux  Outputs=3
  Product : Product
  Product1 : Product
  Sum : Sum  Inputs=+-
  Terminator : Terminator
  Terminator1 : Terminator
  Out1 : Outport
  wires:
  Sum/1 -> Out1/1
  Product1/1 -> Sum/2
  Product/1 -> Sum/1
  Demux/2 -> Terminator1/1
  Demux1/2 -> Terminator/1
  Demux1/3 -> Product1/2  "b3"
  Demux/1 -> Product1/1  "a1"
  Demux1/1 -> Product/2  "b1"
  Demux/3 -> Product/1  "a3"
  A/1 -> Demux/1
  B/1 -> Demux1/1

== system Project_SADC/External torques/SRP torque/Torques on faces of s//c/product vector4/k-component1 ==
  A : Inport
  B : Inport  Port=2
  Demux : Demux  Outputs=3
  Demux1 : Demux  Outputs=3
  Product : Product
  Product1 : Product
  Sum : Sum  Inputs=+-
  Terminator : Terminator
  Terminator1 : Terminator
  Out1 : Outport
  wires:
  Demux/3 -> Terminator1/1  "a3"
  Demux1/3 -> Terminator/1  "b3"
  Demux1/1 -> Product1/2  "b1"
  Demux/2 -> Product1/1  "a2"
  Demux/1 -> Product/1  "a1"
  B/1 -> Demux1/1
  A/1 -> Demux/1
  Demux1/2 -> Product/2  "b2"
  Product/1 -> Sum/1
  Product1/1 -> Sum/2
  Sum/1 -> Out1/1

== system Project_SADC/External torques/SRP torque/Torques on faces of s//c/product vector5/i-component ==
  A : Inport
  B : Inport  Port=2
  Demux : Demux  Outputs=3
  Demux1 : Demux  Outputs=3
  Product : Product
  Product1 : Product
  Sum : Sum  Inputs=+-
  Terminator : Terminator
  Terminator1 : Terminator
  Out2 : Outport
  wires:
  Sum/1 -> Out2/1
  Product1/1 -> Sum/2  "a3b2"
  Demux1/2 -> Product1/2  "b2"
  Product/1 -> Sum/1  "a2b3"
  Demux/2 -> Product/1  "a2"
  Demux/3 -> Product1/1  "a3"
  Demux1/3 -> Product/2  "b3"
  Demux/1 -> Terminator/1  "a1"
  Demux1/1 -> Terminator1/1
  B/1 -> Demux1/1
  A/1 -> Demux/1

== system Project_SADC/External torques/SRP torque/Torques on faces of s//c/product vector5/j-component ==
  A : Inport
  B : Inport  Port=2
  Demux : Demux  Outputs=3
  Demux1 : Demux  Outputs=3
  Product : Product
  Product1 : Product
  Sum : Sum  Inputs=+-
  Terminator : Terminator
  Terminator1 : Terminator
  Out1 : Outport
  wires:
  B/1 -> Demux1/1
  A/1 -> Demux/1
  Demux/3 -> Product/1  "a3"
  Demux1/1 -> Product/2  "b1"
  Demux/1 -> Product1/1  "a1"
  Demux1/3 -> Product1/2  "b3"
  Demux1/2 -> Terminator/1
  Demux/2 -> Terminator1/1
  Product/1 -> Sum/1
  Product1/1 -> Sum/2
  Sum/1 -> Out1/1

== system Project_SADC/External torques/SRP torque/Torques on faces of s//c/product vector5/k-component1 ==
  A : Inport
  B : Inport  Port=2
  Demux : Demux  Outputs=3
  Demux1 : Demux  Outputs=3
  Product : Product
  Product1 : Product
  Sum : Sum  Inputs=+-
  Terminator : Terminator
  Terminator1 : Terminator
  Out1 : Outport
  wires:
  Sum/1 -> Out1/1
  Product1/1 -> Sum/2
  Product/1 -> Sum/1
  Demux1/2 -> Product/2  "b2"
  A/1 -> Demux/1
  B/1 -> Demux1/1
  Demux/1 -> Product/1  "a1"
  Demux/2 -> Product1/1  "a2"
  Demux1/1 -> Product1/2  "b1"
  Demux1/3 -> Terminator/1  "b3"
  Demux/3 -> Terminator1/1  "a3"

== system Project_SADC/External torques/SRP torque/Torques on faces of s//c/product vector6/i-component ==
  A : Inport
  B : Inport  Port=2
  Demux : Demux  Outputs=3
  Demux1 : Demux  Outputs=3
  Product : Product
  Product1 : Product
  Sum : Sum  Inputs=+-
  Terminator : Terminator
  Terminator1 : Terminator
  Out2 : Outport
  wires:
  A/1 -> Demux/1
  B/1 -> Demux1/1
  Demux1/1 -> Terminator1/1
  Demux/1 -> Terminator/1  "a1"
  Demux1/3 -> Product/2  "b3"
  Demux/3 -> Product1/1  "a3"
  Demux/2 -> Product/1  "a2"
  Product/1 -> Sum/1  "a2b3"
  Demux1/2 -> Product1/2  "b2"
  Product1/1 -> Sum/2  "a3b2"
  Sum/1 -> Out2/1

== system Project_SADC/External torques/SRP torque/Torques on faces of s//c/product vector6/j-component ==
  A : Inport
  B : Inport  Port=2
  Demux : Demux  Outputs=3
  Demux1 : Demux  Outputs=3
  Product : Product
  Product1 : Product
  Sum : Sum  Inputs=+-
  Terminator : Terminator
  Terminator1 : Terminator
  Out1 : Outport
  wires:
  Sum/1 -> Out1/1
  Product1/1 -> Sum/2
  Product/1 -> Sum/1
  Demux/2 -> Terminator1/1
  Demux1/2 -> Terminator/1
  Demux1/3 -> Product1/2  "b3"
  Demux/1 -> Product1/1  "a1"
  Demux1/1 -> Product/2  "b1"
  Demux/3 -> Product/1  "a3"
  A/1 -> Demux/1
  B/1 -> Demux1/1

== system Project_SADC/External torques/SRP torque/Torques on faces of s//c/product vector6/k-component1 ==
  A : Inport
  B : Inport  Port=2
  Demux : Demux  Outputs=3
  Demux1 : Demux  Outputs=3
  Product : Product
  Product1 : Product
  Sum : Sum  Inputs=+-
  Terminator : Terminator
  Terminator1 : Terminator
  Out1 : Outport
  wires:
  Demux/3 -> Terminator1/1  "a3"
  Demux1/3 -> Terminator/1  "b3"
  Demux1/1 -> Product1/2  "b1"
  Demux/2 -> Product1/1  "a2"
  Demux/1 -> Product/1  "a1"
  B/1 -> Demux1/1
  A/1 -> Demux/1
  Demux1/2 -> Product/2  "b2"
  Product/1 -> Sum/1
  Product1/1 -> Sum/2
  Sum/1 -> Out1/1

== system Project_SADC/External torques/SRP torque/Torques on faces of s//c/product vector7/i-component ==
  A : Inport
  B : Inport  Port=2
  Demux : Demux  Outputs=3
  Demux1 : Demux  Outputs=3
  Product : Product
  Product1 : Product
  Sum : Sum  Inputs=+-
  Terminator : Terminator
  Terminator1 : Terminator
  Out2 : Outport
  wires:
  Sum/1 -> Out2/1
  Product1/1 -> Sum/2  "a3b2"
  Demux1/2 -> Product1/2  "b2"
  Product/1 -> Sum/1  "a2b3"
  Demux/2 -> Product/1  "a2"
  Demux/3 -> Product1/1  "a3"
  Demux1/3 -> Product/2  "b3"
  Demux/1 -> Terminator/1  "a1"
  Demux1/1 -> Terminator1/1
  B/1 -> Demux1/1
  A/1 -> Demux/1

== system Project_SADC/External torques/SRP torque/Torques on faces of s//c/product vector7/j-component ==
  A : Inport
  B : Inport  Port=2
  Demux : Demux  Outputs=3
  Demux1 : Demux  Outputs=3
  Product : Product
  Product1 : Product
  Sum : Sum  Inputs=+-
  Terminator : Terminator
  Terminator1 : Terminator
  Out1 : Outport
  wires:
  B/1 -> Demux1/1
  A/1 -> Demux/1
  Demux/3 -> Product/1  "a3"
  Demux1/1 -> Product/2  "b1"
  Demux/1 -> Product1/1  "a1"
  Demux1/3 -> Product1/2  "b3"
  Demux1/2 -> Terminator/1
  Demux/2 -> Terminator1/1
  Product/1 -> Sum/1
  Product1/1 -> Sum/2
  Sum/1 -> Out1/1

== system Project_SADC/External torques/SRP torque/Torques on faces of s//c/product vector7/k-component1 ==
  A : Inport
  B : Inport  Port=2
  Demux : Demux  Outputs=3
  Demux1 : Demux  Outputs=3
  Product : Product
  Product1 : Product
  Sum : Sum  Inputs=+-
  Terminator : Terminator
  Terminator1 : Terminator
  Out1 : Outport
  wires:
  Sum/1 -> Out1/1
  Product1/1 -> Sum/2
  Product/1 -> Sum/1
  Demux1/2 -> Product/2  "b2"
  A/1 -> Demux/1
  B/1 -> Demux1/1
  Demux/1 -> Product/1  "a1"
  Demux/2 -> Product1/1  "a2"
  Demux1/1 -> Product1/2  "b1"
  Demux1/3 -> Terminator/1  "b3"
  Demux/3 -> Terminator1/1  "a3"

== system Project_SADC/External torques/SRP torque/Torques on faces of s//c/product vector8/i-component ==
  A : Inport
  B : Inport  Port=2
  Demux : Demux  Outputs=3
  Demux1 : Demux  Outputs=3
  Product : Product
  Product1 : Product
  Sum : Sum  Inputs=+-
  Terminator : Terminator
  Terminator1 : Terminator
  Out2 : Outport
  wires:
  A/1 -> Demux/1
  B/1 -> Demux1/1
  Demux1/1 -> Terminator1/1
  Demux/1 -> Terminator/1  "a1"
  Demux1/3 -> Product/2  "b3"
  Demux/3 -> Product1/1  "a3"
  Demux/2 -> Product/1  "a2"
  Product/1 -> Sum/1  "a2b3"
  Demux1/2 -> Product1/2  "b2"
  Product1/1 -> Sum/2  "a3b2"
  Sum/1 -> Out2/1

== system Project_SADC/External torques/SRP torque/Torques on faces of s//c/product vector8/j-component ==
  A : Inport
  B : Inport  Port=2
  Demux : Demux  Outputs=3
  Demux1 : Demux  Outputs=3
  Product : Product
  Product1 : Product
  Sum : Sum  Inputs=+-
  Terminator : Terminator
  Terminator1 : Terminator
  Out1 : Outport
  wires:
  Sum/1 -> Out1/1
  Product1/1 -> Sum/2
  Product/1 -> Sum/1
  Demux/2 -> Terminator1/1
  Demux1/2 -> Terminator/1
  Demux1/3 -> Product1/2  "b3"
  Demux/1 -> Product1/1  "a1"
  Demux1/1 -> Product/2  "b1"
  Demux/3 -> Product/1  "a3"
  A/1 -> Demux/1
  B/1 -> Demux1/1

== system Project_SADC/External torques/SRP torque/Torques on faces of s//c/product vector8/k-component1 ==
  A : Inport
  B : Inport  Port=2
  Demux : Demux  Outputs=3
  Demux1 : Demux  Outputs=3
  Product : Product
  Product1 : Product
  Sum : Sum  Inputs=+-
  Terminator : Terminator
  Terminator1 : Terminator
  Out1 : Outport
  wires:
  Demux/3 -> Terminator1/1  "a3"
  Demux1/3 -> Terminator/1  "b3"
  Demux1/1 -> Product1/2  "b1"
  Demux/2 -> Product1/1  "a2"
  Demux/1 -> Product/1  "a1"
  B/1 -> Demux1/1
  A/1 -> Demux/1
  Demux1/2 -> Product/2  "b2"
  Product/1 -> Sum/1
  Product1/1 -> Sum/2
  Sum/1 -> Out1/1

== system Project_SADC/External torques/SRP torque/Torques on faces of s//c/product vector9/i-component ==
  A : Inport
  B : Inport  Port=2
  Demux : Demux  Outputs=3
  Demux1 : Demux  Outputs=3
  Product : Product
  Product1 : Product
  Sum : Sum  Inputs=+-
  Terminator : Terminator
  Terminator1 : Terminator
  Out2 : Outport
  wires:
  Sum/1 -> Out2/1
  Product1/1 -> Sum/2  "a3b2"
  Demux1/2 -> Product1/2  "b2"
  Product/1 -> Sum/1  "a2b3"
  Demux/2 -> Product/1  "a2"
  Demux/3 -> Product1/1  "a3"
  Demux1/3 -> Product/2  "b3"
  Demux/1 -> Terminator/1  "a1"
  Demux1/1 -> Terminator1/1
  B/1 -> Demux1/1
  A/1 -> Demux/1

== system Project_SADC/External torques/SRP torque/Torques on faces of s//c/product vector9/j-component ==
  A : Inport
  B : Inport  Port=2
  Demux : Demux  Outputs=3
  Demux1 : Demux  Outputs=3
  Product : Product
  Product1 : Product
  Sum : Sum  Inputs=+-
  Terminator : Terminator
  Terminator1 : Terminator
  Out1 : Outport
  wires:
  B/1 -> Demux1/1
  A/1 -> Demux/1
  Demux/3 -> Product/1  "a3"
  Demux1/1 -> Product/2  "b1"
  Demux/1 -> Product1/1  "a1"
  Demux1/3 -> Product1/2  "b3"
  Demux1/2 -> Terminator/1
  Demux/2 -> Terminator1/1
  Product/1 -> Sum/1
  Product1/1 -> Sum/2
  Sum/1 -> Out1/1

== system Project_SADC/External torques/SRP torque/Torques on faces of s//c/product vector9/k-component1 ==
  A : Inport
  B : Inport  Port=2
  Demux : Demux  Outputs=3
  Demux1 : Demux  Outputs=3
  Product : Product
  Product1 : Product
  Sum : Sum  Inputs=+-
  Terminator : Terminator
  Terminator1 : Terminator
  Out1 : Outport
  wires:
  Sum/1 -> Out1/1
  Product1/1 -> Sum/2
  Product/1 -> Sum/1
  Demux1/2 -> Product/2  "b2"
  A/1 -> Demux/1
  B/1 -> Demux1/1
  Demux/1 -> Product/1  "a1"
  Demux/2 -> Product1/1  "a2"
  Demux1/1 -> Product1/2  "b1"
  Demux1/3 -> Terminator/1  "b3"
  Demux/3 -> Terminator1/1  "a3"

== system Project_SADC/Relative Attitude/DCM from L to B and from L to N/DCM from L to N/Vector norm/norm_vector ==
  u : Inport
  Demux : Demux  Outputs=3
  Square : Math  Operator=square  SaturateOnIntegerOverflow=on
  Square Root : Sqrt  SaturateOnIntegerOverflow=on
  Square1 : Math  Operator=square  SaturateOnIntegerOverflow=on
  Square3 : Math  Operator=square  SaturateOnIntegerOverflow=on
  Sum : Sum  Inputs=+++
  |u| : Outport
  wires:
  u/1 -> Demux/1
  Demux/1 -> Square/1
  Demux/2 -> Square1/1
  Demux/3 -> Square3/1
  Square/1 -> Sum/1
  Square3/1 -> Sum/3
  Square1/1 -> Sum/2
  Sum/1 -> Square Root/1
  Square Root/1 -> |u|/1

== system Project_SADC/Relative Attitude/DCM from L to B and from L to N/DCM from L to N/Vector norm1/norm_vector ==
  u : Inport
  Demux : Demux  Outputs=3
  Square : Math  Operator=square  SaturateOnIntegerOverflow=on
  Square Root : Sqrt  SaturateOnIntegerOverflow=on
  Square1 : Math  Operator=square  SaturateOnIntegerOverflow=on
  Square3 : Math  Operator=square  SaturateOnIntegerOverflow=on
  Sum : Sum  Inputs=+++
  |u| : Outport
  wires:
  u/1 -> Demux/1
  Demux/1 -> Square/1
  Demux/2 -> Square1/1
  Demux/3 -> Square3/1
  Square/1 -> Sum/1
  Square3/1 -> Sum/3
  Square1/1 -> Sum/2
  Sum/1 -> Square Root/1
  Square Root/1 -> |u|/1

== system Project_SADC/Relative Attitude/DCM from L to B and from L to N/DCM from L to N/product vector/i-component ==
  A : Inport
  B : Inport  Port=2
  Demux : Demux  Outputs=3
  Demux1 : Demux  Outputs=3
  Product : Product
  Product1 : Product
  Sum : Sum  Inputs=+-
  Terminator : Terminator
  Terminator1 : Terminator
  Out2 : Outport
  wires:
  Sum/1 -> Out2/1
  Product1/1 -> Sum/2  "a3b2"
  Demux1/2 -> Product1/2  "b2"
  Product/1 -> Sum/1  "a2b3"
  Demux/2 -> Product/1  "a2"
  Demux/3 -> Product1/1  "a3"
  Demux1/3 -> Product/2  "b3"
  Demux/1 -> Terminator/1  "a1"
  Demux1/1 -> Terminator1/1
  B/1 -> Demux1/1
  A/1 -> Demux/1

== system Project_SADC/Relative Attitude/DCM from L to B and from L to N/DCM from L to N/product vector/j-component ==
  A : Inport
  B : Inport  Port=2
  Demux : Demux  Outputs=3
  Demux1 : Demux  Outputs=3
  Product : Product
  Product1 : Product
  Sum : Sum  Inputs=+-
  Terminator : Terminator
  Terminator1 : Terminator
  Out1 : Outport
  wires:
  B/1 -> Demux1/1
  A/1 -> Demux/1
  Demux/3 -> Product/1  "a3"
  Demux1/1 -> Product/2  "b1"
  Demux/1 -> Product1/1  "a1"
  Demux1/3 -> Product1/2  "b3"
  Demux1/2 -> Terminator/1
  Demux/2 -> Terminator1/1
  Product/1 -> Sum/1
  Product1/1 -> Sum/2
  Sum/1 -> Out1/1

== system Project_SADC/Relative Attitude/DCM from L to B and from L to N/DCM from L to N/product vector/k-component1 ==
  A : Inport
  B : Inport  Port=2
  Demux : Demux  Outputs=3
  Demux1 : Demux  Outputs=3
  Product : Product
  Product1 : Product
  Sum : Sum  Inputs=+-
  Terminator : Terminator
  Terminator1 : Terminator
  Out1 : Outport
  wires:
  Sum/1 -> Out1/1
  Product1/1 -> Sum/2
  Product/1 -> Sum/1
  Demux1/2 -> Product/2  "b2"
  A/1 -> Demux/1
  B/1 -> Demux1/1
  Demux/1 -> Product/1  "a1"
  Demux/2 -> Product1/1  "a2"
  Demux1/1 -> Product1/2  "b1"
  Demux1/3 -> Terminator/1  "b3"
  Demux/3 -> Terminator1/1  "a3"

== matlab function Project_SADC/Attitude determination /A determination/A_det ==
  data: A output; mag_s input; Sun_s input; Earth_s input; mag_N input; Sun_N input; Earth_N input; weights input; c output; wb_sens input; A_prev input; A_dot output
function [A,c,A_dot]  = fcn(mag_s,Sun_s,Earth_s,mag_N,Sun_N,Earth_N,weights,wb_sens,A_prev)
 
if (Sun_s == zeros(3,1) & Earth_s ~= zeros(3,1))
% TRIAD
    s1 = Earth_s;
    s2 = cross(Earth_s,mag_s)/norm(cross(Earth_s,mag_s));
    s3 = cross(s1,s2);
    v1 = Earth_N;
    v2 = cross(Earth_N,mag_N)/norm(cross(Earth_N,mag_N));
    v3 = cross(v1,v2);
    S = [s1 s2 s3];
    V = [v1 v2 v3]; 
    A = S*V';
    A_dot = zeros(3);
    c =-1; 

elseif (Sun_s == zeros(3,1) & Earth_s == zeros(3,1))
   
    w_skew = [0 -wb_sens(3) wb_sens(2); wb_sens(3) 0 -wb_sens(1);-wb_sens(2) wb_sens(1) 0];
    A_dot = -w_skew*A_prev; 
    c = 2;
    A = zeros(3);

else
    b = [mag_s , Sun_s , Earth_s];
    r = [mag_N , Sun_N , Earth_N];
    B = weights(1)*mag_s*mag_N'+ weights(2)*Sun_s*Sun_N'+weights(3)*Earth_s*Earth_N';
    [U,S,V] = svd(B);
    d = det(U)*det(V);
    A = U * diag([1,1,d])*V';
    c = -3;
    A_dot = zeros(3);

end


end
